simulink model "Run"  (R2024a)
settings: Solver=VariableStepAuto  StartTime=0.0  StopTime=20  RelTol=1e-3
settings Model: Creator=patwa  LastModifiedBy=patwa

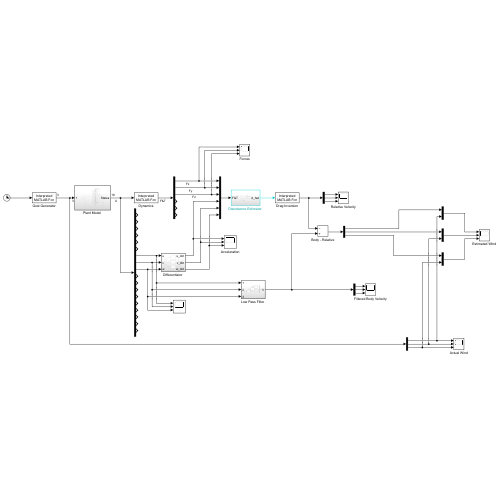
[thumbnail: Simulink's stored preview of the top-level diagram]
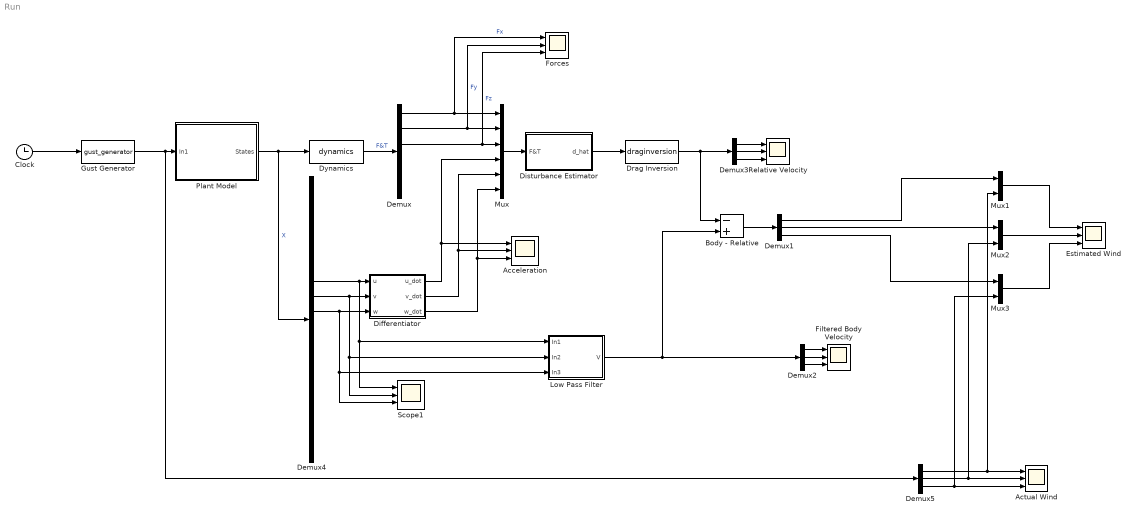
== system Run ==
  Acceleration : Scope  NumInputPorts=3
  Actual Wind : Scope  NumInputPorts=3
  Body - Relative : Sum  Inputs=-+
  Clock : Clock
  Demux : Demux  Outputs=6
  Demux{1..3,5} (4 alike) : Demux  Outputs=3
  Demux4 : Demux  Outputs=18
  "Differentiator " : Subsystem
  "Disturbance Estimator " : Subsystem
  Drag Inversion : MATLABFcn  MATLABFcn=draginversion  OutputDimensions=3
  Dynamics : MATLABFcn  MATLABFcn=dynamics  OutputDimensions=6
  Estimated Wind : Scope  NumInputPorts=3
  Filtered Body Velocity : Scope  NumInputPorts=3
  Forces : Scope  NumInputPorts=3
  Gust Generator : MATLABFcn  MATLABFcn=gust_generator
  "Low Pass Filter " : Subsystem
  Mux : Mux  Inputs=6
  Mux1 : Mux  Inputs=2
  Mux2 : Mux  Inputs=2
  Mux3 : Mux  Inputs=2
  "Plant Model " : Subsystem
  Relative Velocity : Scope  NumInputPorts=3
  Scope1 : Scope  NumInputPorts=3
  wires:
  Dynamics/1 -> Demux/1  "F&T"
  Demux/1 -> Forces/1, Mux/1  "Fx"
  Demux/2 -> Mux/2, Forces/2  "Fy"
  Demux/3 -> Forces/3, Mux/3  "Fz"
  Mux/1 -> "Disturbance Estimator "/1(F&T)
  "Disturbance Estimator "/1(d_hat) -> Drag Inversion/1
  "Differentiator "/1(u_dot) -> Acceleration/1, Mux/4
  "Differentiator "/2(v_dot) -> Acceleration/2, Mux/5
  "Differentiator "/3(w_dot) -> Acceleration/3, Mux/6
  Body - Relative/1 -> Demux1/1
  Demux2/3 -> Filtered Body Velocity/3
  Demux2/2 -> Filtered Body Velocity/2
  Demux2/1 -> Filtered Body Velocity/1
  "Low Pass Filter "/1(V) -> Demux2/1, Body - Relative/2
  Demux3/3 -> Relative Velocity/3
  Demux3/2 -> Relative Velocity/2
  Demux3/1 -> Relative Velocity/1
  Drag Inversion/1 -> Demux3/1, Body - Relative/1
  Clock/1 -> Gust Generator/1
  Gust Generator/1 -> Demux5/1, "Plant Model "/1(In1)
  "Plant Model "/1(States) -> Demux4/1, Dynamics/1  "X"
  Demux4/7 -> "Low Pass Filter "/1(In1), Scope1/1, "Differentiator "/1(u)
  Demux4/8 -> "Differentiator "/2(v), "Low Pass Filter "/2(In2), Scope1/2
  Demux4/9 -> "Differentiator "/3(w), Scope1/3, "Low Pass Filter "/3(In3)
  Demux5/1 -> Mux1/2, Actual Wind/1
  Demux5/2 -> Actual Wind/2, Mux2/2
  Demux5/3 -> Mux3/2, Actual Wind/3
  Demux1/1 -> Mux1/1
  Demux1/2 -> Mux2/1
  Demux1/3 -> Mux3/1
  Mux1/1 -> Estimated Wind/1
  Mux2/1 -> Estimated Wind/2
  Mux3/1 -> Estimated Wind/3

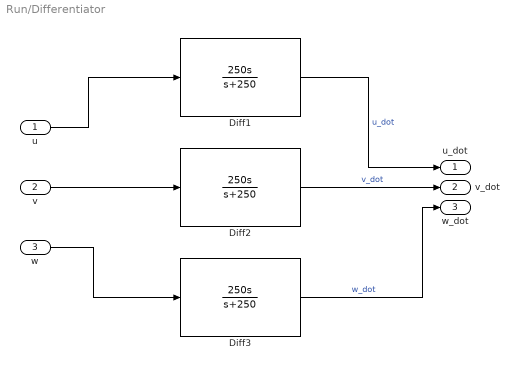
== system Run/Differentiator  ==
  u : Inport
  v : Inport  Port=2
  w : Inport  Port=3
  Diff1 : TransferFcn  Numerator=[250 0]  Denominator=[1 250]
  Diff2 : TransferFcn  Numerator=[250 0]  Denominator=[1 250]
  Diff3 : TransferFcn  Numerator=[250 0]  Denominator=[1 250]
  u_dot : Outport
  v_dot : Outport  Port=2
  w_dot : Outport  Port=3
  wires:
  v/1 -> Diff2/1
  Diff3/1 -> w_dot/1  "w_dot"
  u/1 -> Diff1/1
  Diff1/1 -> u_dot/1  "u_dot"
  w/1 -> Diff3/1
  Diff2/1 -> v_dot/1  "v_dot"

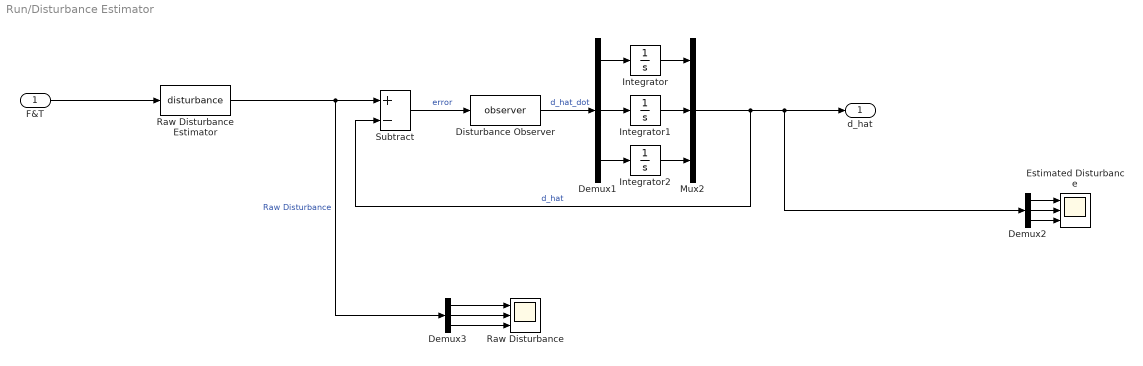
== system Run/Disturbance Estimator  ==
  F&T : Inport
  Demux1 : Demux  Outputs=3
  Demux2 : Demux  Outputs=3
  Demux3 : Demux  Outputs=3
  Disturbance Observer : MATLABFcn  MATLABFcn=observer  OutputDimensions=3
  Estimated Disturbance : Scope  NumInputPorts=3
  Integrator : Integrator
  Integrator1 : Integrator
  Integrator2 : Integrator
  Mux2 : Mux  Inputs=3
  Raw Disturbance : Scope  NumInputPorts=3
  Raw Disturbance Estimator : MATLABFcn  MATLABFcn=disturbance  OutputDimensions=3
  Subtract : Sum  Inputs=+-
  d_hat : Outport
  wires:
  Integrator2/1 -> Mux2/3
  Demux1/1 -> Integrator/1
  Demux1/2 -> Integrator1/1
  Subtract/1 -> Disturbance Observer/1  "error"
  Disturbance Observer/1 -> Demux1/1  "d_hat_dot"
  Demux1/3 -> Integrator2/1
  F&T/1 -> Raw Disturbance Estimator/1
  Integrator1/1 -> Mux2/2
  Integrator/1 -> Mux2/1
  Mux2/1 -> Subtract/2, Demux2/1, d_hat/1  "d_hat"
  Demux2/1 -> Estimated Disturbance/1
  Demux2/2 -> Estimated Disturbance/2
  Demux2/3 -> Estimated Disturbance/3
  Demux3/2 -> Raw Disturbance/2
  Demux3/1 -> Raw Disturbance/1
  Raw Disturbance Estimator/1 -> Demux3/1, Subtract/1  "Raw Disturbance"
  Demux3/3 -> Raw Disturbance/3

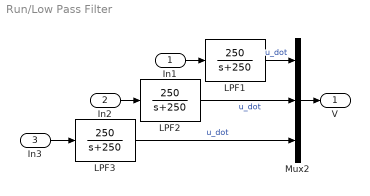
== system Run/Low Pass Filter  ==
  In1 : Inport
  In2 : Inport  Port=2
  In3 : Inport  Port=3
  LPF1 : TransferFcn  Numerator=[250]  Denominator=[1 250]
  LPF2 : TransferFcn  Numerator=[250]  Denominator=[1 250]
  LPF3 : TransferFcn  Numerator=[250]  Denominator=[1 250]
  Mux2 : Mux  Inputs=3
  V : Outport
  wires:
  LPF2/1 -> Mux2/2  "u_dot"
  LPF1/1 -> Mux2/1  "u_dot"
  In3/1 -> LPF3/1
  Mux2/1 -> V/1
  LPF3/1 -> Mux2/3  "u_dot"
  In2/1 -> LPF2/1
  In1/1 -> LPF1/1

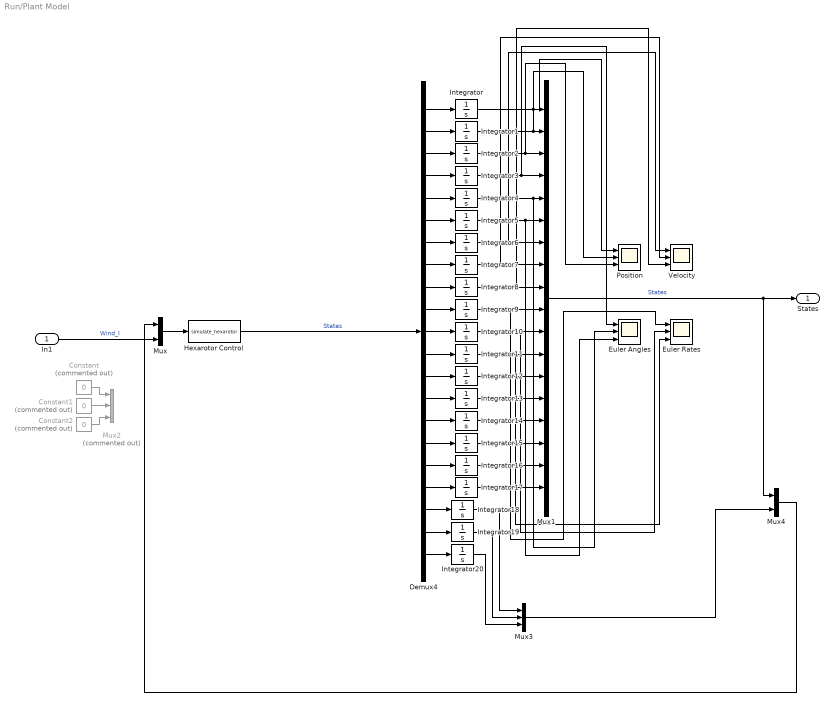
== system Run/Plant Model  ==
  In1 : Inport
  Constant : Constant  Commented=on  Value=0
  Constant1 : Constant  Commented=on  Value=0
  Constant2 : Constant  Commented=on  Value=0
  Demux4 : Demux  Outputs=21
  Euler Angles : Scope  NumInputPorts=3
  Euler Rates : Scope  NumInputPorts=3
  Hexarotor Control : MATLABFcn  MATLABFcn=simulate_hexarotor  OutputDimensions=21
  Integrator{,1..20} (21 alike) : Integrator
  Mux : Mux  Inputs=2
  Mux1 : Mux  Inputs=18
  Mux2 : Mux  Commented=on  Inputs=3
  Mux3 : Mux  Inputs=3
  Mux4 : Mux  Inputs=2
  Position : Scope  NumInputPorts=3
  Velocity : Scope  NumInputPorts=3
  States : Outport
  wires:
  Demux4/12 -> Integrator11/1
  Demux4/17 -> Integrator16/1
  Demux4/13 -> Integrator12/1
  Demux4/15 -> Integrator14/1
  Hexarotor Control/1 -> Demux4/1  "States"
  Demux4/14 -> Integrator13/1
  Demux4/1 -> Integrator/1
  Demux4/7 -> Integrator6/1
  Demux4/6 -> Integrator5/1
  Demux4/18 -> Integrator17/1
  Demux4/10 -> Integrator9/1
  Demux4/5 -> Integrator4/1
  Demux4/3 -> Integrator2/1
  Demux4/8 -> Integrator7/1
  Demux4/4 -> Integrator3/1
  Demux4/2 -> Integrator1/1
  Demux4/11 -> Integrator10/1
  Demux4/9 -> Integrator8/1
  Demux4/16 -> Integrator15/1
  Mux1/1 -> Mux4/1, States/1  "States"
  Integrator/1 -> Position/1, Mux1/1
  Integrator1/1 -> Position/2, Mux1/2
  Integrator2/1 -> Mux1/3, Position/3
  Integrator3/1 -> Mux1/4, Euler Angles/1
  Integrator4/1 -> Euler Angles/2, Mux1/5
  Integrator5/1 -> Mux1/6, Euler Angles/3
  Integrator6/1 -> Mux1/7, Velocity/1
  Integrator7/1 -> Mux1/8, Velocity/2
  Integrator8/1 -> Mux1/9, Velocity/3
  Integrator9/1 -> Mux1/10, Euler Rates/1
  Integrator10/1 -> Mux1/11, Euler Rates/2
  Integrator11/1 -> Mux1/12, Euler Rates/3
  Integrator12/1 -> Mux1/13
  Integrator13/1 -> Mux1/14
  Integrator14/1 -> Mux1/15
  Integrator15/1 -> Mux1/16
  Integrator16/1 -> Mux1/17
  Integrator17/1 -> Mux1/18
  Mux/1 -> Hexarotor Control/1
  Constant1/1 -> Mux2/2
  Constant/1 -> Mux2/1
  Constant2/1 -> Mux2/3
  In1/1 -> Mux/2  "Wind_I"
  Demux4/19 -> Integrator18/1
  Demux4/20 -> Integrator19/1
  Demux4/21 -> Integrator20/1
  Integrator19/1 -> Mux3/2
  Integrator18/1 -> Mux3/1
  Integrator20/1 -> Mux3/3
  Mux3/1 -> Mux4/2
  Mux4/1 -> Mux/1
